simulink model "twolevel_seriesparallel"  (R2016a)
settings: Solver=VariableStepAuto  StartTime=0.0  StopTime=stop_time  RelTol=1e-3  AbsTol=1e-6
values from neighbouring files (symbols this model uses):
  DCLINK_Cap = 0.65*1.35*capacitorsabiti/sw_frequency    (= 0.000406115702479)    [loadvariation.m]    (also in trials.m = 1.35*capacitorsabiti/sw_frequency; twolevel_seriesparallel_analysis.m)
  Ef = Vln_rms*cos(Load_Angle)    [loadvariation.m]    (also in trials.m; twolevel_seriesparallel_analysis.m)
  intangle1 = 0    [loadvariation.m]    (also in trials.m; twolevel_seriesparallel_analysis.m)
  intangle2 = interleaving_angle    (= 180)    [loadvariation.m]    (also in trials.m = 360; twolevel_seriesparallel_analysis.m)
  intangle3 = 0    [loadvariation.m]    (also in trials.m; twolevel_seriesparallel_analysis.m)
  intangle4 = interleaving_angle    (= 180)    [loadvariation.m]    (also in trials.m = 360; twolevel_seriesparallel_analysis.m)
  Load_Angle = acos(Load_Power_Factor)    [loadvariation.m]    (also in trials.m; twolevel_seriesparallel_analysis.m)
  Ls = n*m*Xs/ref_frequency    [loadvariation.m]    (also in trials.m; twolevel_seriesparallel_analysis.m)
  ma = 0.9    [loadvariation.m]    (also in trials.m; twolevel_seriesparallel_analysis.m)
  ref_frequency = 2*pi*50    (= 314.159265359)    [loadvariation.m]    (also in trials.m; twolevel_seriesparallel_analysis.m)
  Sampling_time = 1/(100*sw_frequency)    (= 1.65289256198e-06)    [loadvariation.m]    (also in twolevel_seriesparallel_analysis.m = 8.26446280992e-06)
  Vin = DC_Voltage_Source + Rin*(Load_Real_Power/DC_Voltage_Source)    (= 554.814814815)    [loadvariation.m]    (also in trials.m; twolevel_seriesparallel_analysis.m)
undefined symbols (not defined in the file or in its folder): intangle5, intangle6, intangle7, intangle8, Lload, Rload
libraries: powerlib x106, powerlib_meascontrol x58, simulink x24
(part 1 of 2)
settings Model: Creator=hakan  LastModifiedBy=hakan
settings DataIOCC: SaveState=on
settings DebuggingCC: UnconnectedInputMsg=none  UnconnectedOutputMsg=none  UnconnectedLineMsg=none

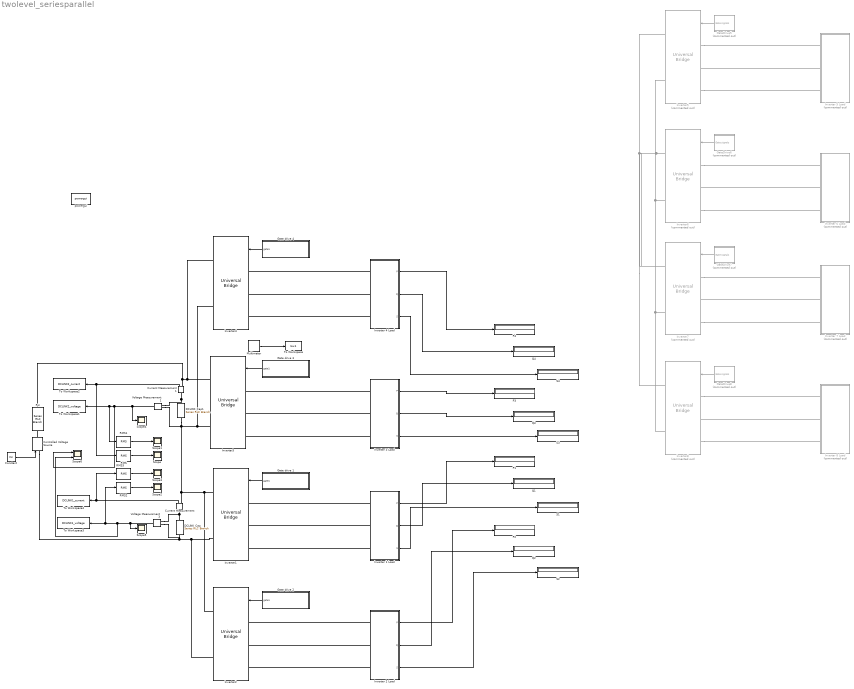
== system twolevel_seriesparallel ==
  Constant : Constant  Value=Vin
  Controlled Voltage Source : powerlib/Electrical Sources/Controlled Voltage Source  Initialize=on  Source_Type=AC  Amplitude=0  Phase=0  Frequency=0  Measurements=None
  Current Measurement : powerlib/Measurements/Current Measurement  PhasorSimulation=off  OutputType=Complex  PSBequivalent=0
  Current Measurement1 : powerlib/Measurements/Current Measurement  PhasorSimulation=off  OutputType=Complex  PSBequivalent=0
  DCLINK_Cap : powerlib/Elements/Series RLC Branch  LConnTagsString=__new0  RConnTagsString=__new0  BranchType=C  Resistance=1  Inductance=1e-3  SetiL0=off  InitialCurrent=0  Capacitance=DCLINK_Cap  Setx0=on  InitialVoltage=270  Measurements=None
  DCLINK_Cap1 : powerlib/Elements/Series RLC Branch  LConnTagsString=__new0  RConnTagsString=__new0  BranchType=C  Resistance=1  Inductance=1e-3  SetiL0=off  InitialCurrent=0  Capacitance=DCLINK_Cap  Setx0=on  InitialVoltage=270  Measurements=None
  Gate drive 1 : Subsystem
  Gate drive 2 : Subsystem
  Gate drive 3 : Subsystem
  Gate drive 4 : Subsystem
  GateDrive5 : Subsystem  Commented=on
  GateDrive6 : Subsystem  Commented=on
  GateDrive7 : Subsystem  Commented=on
  GateDrive8 : Subsystem  Commented=on
  Inverter 1 Load : Subsystem
  Inverter 2 Load : Subsystem
  Inverter 3 Load : Subsystem
  Inverter 4 Load : Subsystem
  Inverter 5 Load : Subsystem  Commented=on
  Inverter 6 Load : Subsystem  Commented=on
  Inverter 7 Load : Subsystem  Commented=on
  Inverter 8 Load : Subsystem  Commented=on
  Inverter1 : powerlib/Power Electronics/Universal Bridge  Arms=3  SnubberResistance=1e5  SnubberCapacitance=inf  Device=IGBT / Diodes  Ron=1e-3  Lon=0  ForwardVoltages="[  0  0  ]"  ForwardVoltage=0  GTOparameters=[ 10e-6 , 20e-6 ]  IGBTparameters=[ 1e-6 , 2e-6 ]  Measurements=None  Measurements_2=None  converterType=Rectifier
  Inverter2 : powerlib/Power Electronics/Universal Bridge  Arms=3  SnubberResistance=1e5  SnubberCapacitance=inf  Device=IGBT / Diodes  Ron=1e-3  Lon=0  ForwardVoltages="[  0  0  ]"  ForwardVoltage=0  GTOparameters=[ 10e-6 , 20e-6 ]  IGBTparameters=[ 1e-6 , 2e-6 ]  Measurements=None  Measurements_2=None  converterType=Rectifier
  Inverter3 : powerlib/Power Electronics/Universal Bridge  Arms=3  SnubberResistance=1e5  SnubberCapacitance=inf  Device=IGBT / Diodes  Ron=1e-3  Lon=0  ForwardVoltages="[  0  0  ]"  ForwardVoltage=0  GTOparameters=[ 10e-6 , 20e-6 ]  IGBTparameters=[ 1e-6 , 2e-6 ]  Measurements=All voltages and currents  Measurements_2=None  converterType=Rectifier
  Inverter4 : powerlib/Power Electronics/Universal Bridge  Arms=3  SnubberResistance=1e5  SnubberCapacitance=inf  Device=IGBT / Diodes  Ron=1e-3  Lon=0  ForwardVoltages="[  0  0  ]"  ForwardVoltage=0  GTOparameters=[ 10e-6 , 20e-6 ]  IGBTparameters=[ 1e-6 , 2e-6 ]  Measurements=None  Measurements_2=None  converterType=Rectifier
  Inverter{5..8} (4 alike) : powerlib/Power Electronics/Universal Bridge  Commented=on  Arms=3  SnubberResistance=1e5  SnubberCapacitance=inf  Device=IGBT / Diodes  Ron=1e-3  Lon=0  ForwardVoltages="[  0  0  ]"  ForwardVoltage=0  GTOparameters=[ 10e-6 , 20e-6 ]  IGBTparameters=[ 1e-6 , 2e-6 ]  Measurements=None  Measurements_2=None  converterType=Rectifier
  Multimeter : powerlib/Measurements/Multimeter  PhasorSimulation=off  OutputType=Complex  sel=11  L=16  Gain=1  yselected={'Isw1: Inverter3'};  PSBOutputType=1  PSBequivalent=0  AxesSetting=[0,0.1,-100,100]  Display=0  SavedBlockNames=-11
  P{1..4} (4 alike) : Display
  Q{1..4} (4 alike) : Display
  RMS{,1..3} (4 alike) : powerlib_meascontrol/Measurements/RMS  TrueRMS=on  Freq=Load_Nominal_Freq  RMSInit=10  Ts=0
  Rin : powerlib/Elements/Series RLC Branch  LConnTagsString=__new0  RConnTagsString=__new0  BranchType=R  Resistance=1  Inductance=1e-3  SetiL0=off  InitialCurrent=0  Capacitance=1000e-6  Setx0=off  InitialVoltage=0  Measurements=None
  S{1..4} (4 alike) : Display
  Scope{,1..5} (6 alike) : Scope
  Scope6 : Scope  NumInputPorts=2
  To Workspace : ToWorkspace  VariableName=Isw1  SaveFormat=Structure With Time  SampleTime=-1
  To Workspace1 : ToWorkspace  VariableName=DCLINK2_voltage  SaveFormat=Structure With Time  SampleTime=-1
  To Workspace2 : ToWorkspace  VariableName=DCLINK2_current  SaveFormat=Structure With Time  SampleTime=-1
  To Workspace3 : ToWorkspace  VariableName=DCLINK1_voltage  SaveFormat=Structure With Time  SampleTime=-1
  To Workspace4 : ToWorkspace  VariableName=DCLINK1_current  SaveFormat=Structure With Time  SampleTime=-1
  Voltage Measurement1 : powerlib/Measurements/Voltage Measurement  PhasorSimulation=off  OutputType=Complex  PSBequivalent=0
  Voltage Measurement3 : powerlib/Measurements/Voltage Measurement  PhasorSimulation=off  OutputType=Complex  PSBequivalent=0
  powergui : powerlib/powergui  Priority=1  SimulationMode=Discrete  SolverType=Tustin/Backward Euler (TBE)  SampleTime=Sampling_time  frequency=60  SPID=off  DisableSnubberDevices=off  DisableRonSwitches=off  DisableVfSwitches=off  SwTol=0  DisplayEquations=off  Interpol=off  ExternalGateDelay=off  methode=off  Ts=10  FunctionMessages=off  echomessages=off  HookPort=off  EnableUseOfTLC=off  x0status=blocks  frequencyindice=0  Pbase=100e6  ErrMax=1e-4  Iterations=50  UnitsV=kV  UnitsW=MW  buscounter=0  RestoreLinks=warning  ResistiveCurrentMeasurement=off  Frange=[0:2:500]  Ylog=off  Xlog=on  ShowGrid=off  save=off  variable=ZData  structure=DCLINK1_current  ZoomFFT=off  StartTime=0  cycles=35  DisplayStyle=4  fundamental=50  FreqAxis=off  MaxFrequency=300000  frequencyindicesteady=1  RmsSteady=1  display=off
  wires:
  Constant/1 -> Controlled Voltage Source/1
  Gate drive 1/1(gate1) -> Inverter1/1
  Current Measurement/1 -> RMS3/1, To Workspace4/1
  Gate drive 2/1(gate1) -> Inverter2/1
  GateDrive5/1(Gate signals) -> Inverter5/1
  GateDrive6/1(Gate signals) -> Inverter6/1
  GateDrive7/1(Gate signals) -> Inverter7/1
  GateDrive8/1(Gate signals) -> Inverter8/1
  Current Measurement1/1 -> RMS/1, To Workspace2/1
  Voltage Measurement1/1 -> Scope4/1, Scope6/1, RMS1/1, To Workspace1/1
  RMS/1 -> Scope/1
  RMS1/1 -> Scope1/1
  RMS2/1 -> Scope2/1
  RMS3/1 -> Scope3/1
  Voltage Measurement3/1 -> Scope6/2, RMS2/1, To Workspace3/1, Scope5/1
  Gate drive 4/1(gate1) -> Inverter4/1
  Gate drive 3/1(gate1) -> Inverter3/1
  Inverter 1 Load/2(Q) -> Q1/1
  Inverter 1 Load/3(S) -> S1/1
  Inverter 2 Load/1(P) -> P2/1
  Inverter 2 Load/2(Q) -> Q2/1
  Inverter 2 Load/3(S) -> S2/1
  Inverter 1 Load/1(P) -> P1/1
  Inverter 4 Load/2(Q) -> Q4/1
  Inverter 4 Load/3(S) -> S4/1
  Inverter 3 Load/1(P) -> P3/1
  Inverter 3 Load/2(Q) -> Q3/1
  Inverter 3 Load/3(S) -> S3/1
  Inverter 4 Load/1(P) -> P4/1
  Multimeter/1 -> To Workspace/1
  connections:
  Voltage Measurement3/LConn1 -- Current Measurement/LConn1 -- DCLINK_Cap/LConn1
  Inverter 1 Load/LConn3 -- Inverter1/LConn3
  Inverter 1 Load/LConn1 -- Inverter1/LConn1
  Controlled Voltage Source/RConn1 -- Rin/RConn1
  Inverter 2 Load/LConn2 -- Inverter2/LConn2
  Inverter 1 Load/LConn2 -- Inverter1/LConn2
  Inverter 2 Load/LConn1 -- Inverter2/LConn1
  Inverter 2 Load/LConn3 -- Inverter2/LConn3
  Inverter 3 Load/LConn1 -- Inverter3/LConn1
  Inverter 4 Load/LConn3 -- Inverter4/LConn3
  Inverter 3 Load/LConn3 -- Inverter3/LConn3
  Inverter 3 Load/LConn2 -- Inverter3/LConn2
  Inverter 4 Load/LConn1 -- Inverter4/LConn1
  Inverter 4 Load/LConn2 -- Inverter4/LConn2
  Inverter7/LConn3 -- Inverter 7 Load/LConn3
  Inverter6/LConn3 -- Inverter 6 Load/LConn3
  Inverter5/LConn1 -- Inverter 5 Load/LConn1
  Inverter 5 Load/LConn2 -- Inverter5/LConn2
  Inverter8/LConn3 -- Inverter 8 Load/LConn3
  Inverter5/LConn3 -- Inverter 5 Load/LConn3
  Inverter7/LConn1 -- Inverter 7 Load/LConn1
  Inverter6/LConn1 -- Inverter 6 Load/LConn1
  Inverter 8 Load/LConn2 -- Inverter8/LConn2
  Inverter 6 Load/LConn2 -- Inverter6/LConn2
  Inverter8/LConn1 -- Inverter 8 Load/LConn1
  Inverter 7 Load/LConn2 -- Inverter7/LConn2
  DCLINK_Cap1/LConn1 -- Current Measurement1/LConn1 -- Voltage Measurement1/LConn1
  Inverter8/RConn2 -- Inverter5/RConn2 -- Inverter6/RConn2 -- Inverter7/RConn2
  Inverter6/RConn1 -- Inverter8/RConn1 -- Inverter7/RConn1 -- Inverter5/RConn1
  Current Measurement1/RConn1 -- Rin/LConn1 -- Inverter4/RConn1 -- Inverter3/RConn1
  Inverter2/RConn2 -- Inverter1/RConn2 -- Controlled Voltage Source/LConn1 -- DCLINK_Cap/RConn1 -- Voltage Measurement3/LConn2
  Voltage Measurement1/LConn2 -- Inverter4/RConn2 -- Inverter3/RConn2 -- DCLINK_Cap1/RConn1 -- Current Measurement/RConn1 -- Inverter2/RConn1 -- Inverter1/RConn1

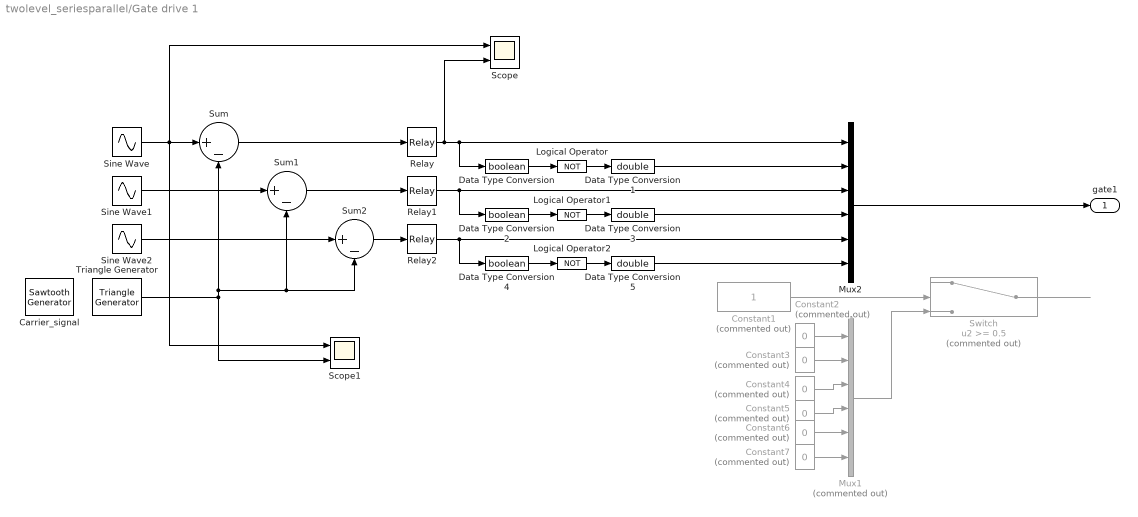
== system twolevel_seriesparallel/Gate drive 1 ==
  Carrier_signal : powerlib_meascontrol/Pulse & Signal Generators/Sawtooth Generator  Freq=sw_frequency  Phase=intangle1  Ts=0
  Constant1 : Constant  Commented=on
  Constant{2..7} (6 alike) : Constant  Commented=on  Value=0
  Data Type Conversion : DataTypeConversion  OutDataTypeStr=boolean
  Data Type Conversion1 : DataTypeConversion  OutDataTypeStr=double
  Data Type Conversion2 : DataTypeConversion  OutDataTypeStr=boolean
  Data Type Conversion3 : DataTypeConversion  OutDataTypeStr=double
  Data Type Conversion4 : DataTypeConversion  OutDataTypeStr=boolean
  Data Type Conversion5 : DataTypeConversion  OutDataTypeStr=double
  Logical Operator : Logic  Operator=NOT  AllPortsSameDT=off  OutDataTypeStr=boolean
  Logical Operator1 : Logic  Operator=NOT  AllPortsSameDT=off  OutDataTypeStr=boolean
  Logical Operator2 : Logic  Operator=NOT  AllPortsSameDT=off  OutDataTypeStr=boolean
  Mux1 : Mux  Commented=on  Inputs=6
  Mux2 : Mux  Inputs=6
  Relay : Relay
  Relay1 : Relay
  Relay2 : Relay
  Scope : Scope  NumInputPorts=2
  Scope1 : Scope  NumInputPorts=2
  Sine Wave : Sin  Amplitude=ma  Frequency=ref_frequency  Phase=Load_Angle  SampleTime=0
  Sine Wave1 : Sin  Amplitude=ma  Frequency=ref_frequency  Phase=-2*pi/3+Load_Angle  SampleTime=0
  Sine Wave2 : Sin  Amplitude=ma  Frequency=ref_frequency  Phase=2*pi/3+Load_Angle  SampleTime=0
  Sum : Sum  Inputs=|+-
  Sum1 : Sum  Inputs=|+-
  Sum2 : Sum  Inputs=|+-
  Switch : Switch  Commented=on  Threshold=0.5
  Triangle Generator : powerlib_meascontrol/Pulse & Signal Generators/Triangle Generator  Freq=sw_frequency  Phase=intangle1  Ts=0
  gate1 : Outport
  wires:
  Sine Wave/1 -> Scope1/1, Scope/1, Sum/1
  Triangle Generator/1 -> Sum1/2, Sum2/2, Sum/2, Scope1/2
  Sine Wave1/1 -> Sum1/1
  Sine Wave2/1 -> Sum2/1
  Sum/1 -> Relay/1
  Sum1/1 -> Relay1/1
  Sum2/1 -> Relay2/1
  Data Type Conversion/1 -> Logical Operator/1
  Relay/1 -> Scope/2, Data Type Conversion/1, Mux2/1
  Logical Operator/1 -> Data Type Conversion1/1
  Data Type Conversion1/1 -> Mux2/2
  Data Type Conversion2/1 -> Logical Operator1/1
  Relay1/1 -> Data Type Conversion2/1, Mux2/3
  Logical Operator1/1 -> Data Type Conversion3/1
  Data Type Conversion3/1 -> Mux2/4
  Data Type Conversion4/1 -> Logical Operator2/1
  Relay2/1 -> Data Type Conversion4/1, Mux2/5
  Logical Operator2/1 -> Data Type Conversion5/1
  Data Type Conversion5/1 -> Mux2/6
  Constant1/1 -> Switch/2
  Constant2/1 -> Mux1/1
  Constant3/1 -> Mux1/2
  Constant4/1 -> Mux1/3
  Constant5/1 -> Mux1/4
  Constant7/1 -> Mux1/6
  Constant6/1 -> Mux1/5
  Mux1/1 -> Switch/3
  Switch/1 -> ?
  Mux2/1 -> gate1/1

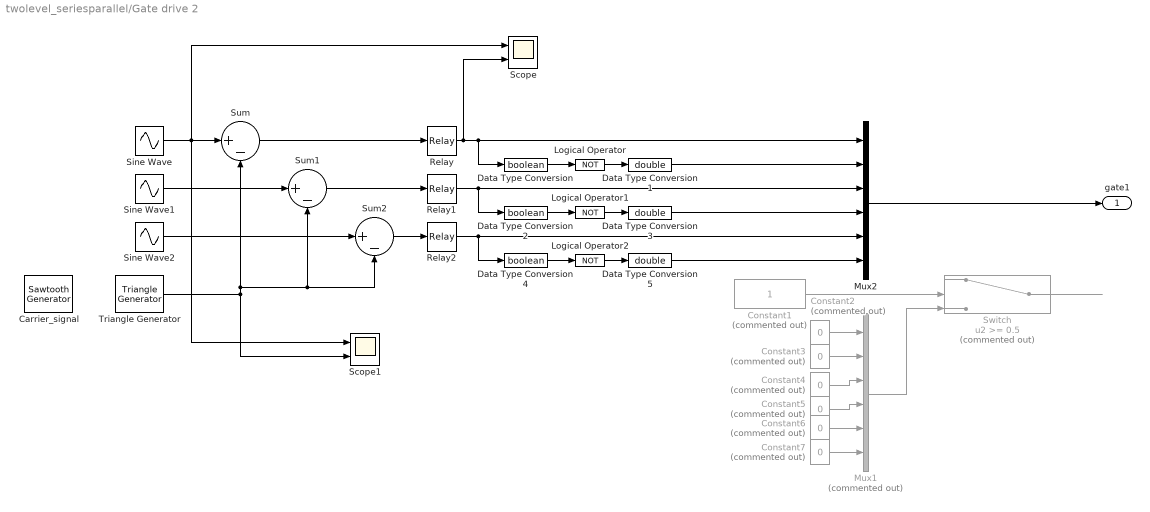
== system twolevel_seriesparallel/Gate drive 2 ==
  Carrier_signal : powerlib_meascontrol/Pulse & Signal Generators/Sawtooth Generator  Freq=sw_frequency  Phase=intangle2  Ts=0
  Constant1 : Constant  Commented=on
  Constant{2..7} (6 alike) : Constant  Commented=on  Value=0
  Data Type Conversion : DataTypeConversion  OutDataTypeStr=boolean
  Data Type Conversion1 : DataTypeConversion  OutDataTypeStr=double
  Data Type Conversion2 : DataTypeConversion  OutDataTypeStr=boolean
  Data Type Conversion3 : DataTypeConversion  OutDataTypeStr=double
  Data Type Conversion4 : DataTypeConversion  OutDataTypeStr=boolean
  Data Type Conversion5 : DataTypeConversion  OutDataTypeStr=double
  Logical Operator : Logic  Operator=NOT  AllPortsSameDT=off  OutDataTypeStr=boolean
  Logical Operator1 : Logic  Operator=NOT  AllPortsSameDT=off  OutDataTypeStr=boolean
  Logical Operator2 : Logic  Operator=NOT  AllPortsSameDT=off  OutDataTypeStr=boolean
  Mux1 : Mux  Commented=on  Inputs=6
  Mux2 : Mux  Inputs=6
  Relay : Relay
  Relay1 : Relay
  Relay2 : Relay
  Scope : Scope  NumInputPorts=2
  Scope1 : Scope  NumInputPorts=2
  Sine Wave : Sin  Amplitude=ma  Frequency=ref_frequency  Phase=Load_Angle  SampleTime=0
  Sine Wave1 : Sin  Amplitude=ma  Frequency=ref_frequency  Phase=-2*pi/3+Load_Angle  SampleTime=0
  Sine Wave2 : Sin  Amplitude=ma  Frequency=ref_frequency  Phase=2*pi/3+Load_Angle  SampleTime=0
  Sum : Sum  Inputs=|+-
  Sum1 : Sum  Inputs=|+-
  Sum2 : Sum  Inputs=|+-
  Switch : Switch  Commented=on  Threshold=0.5
  Triangle Generator : powerlib_meascontrol/Pulse & Signal Generators/Triangle Generator  Freq=sw_frequency  Phase=intangle2  Ts=0
  gate1 : Outport
  wires:
  Sine Wave/1 -> Scope1/1, Scope/1, Sum/1
  Triangle Generator/1 -> Sum1/2, Sum2/2, Sum/2, Scope1/2
  Sine Wave1/1 -> Sum1/1
  Sine Wave2/1 -> Sum2/1
  Sum/1 -> Relay/1
  Sum1/1 -> Relay1/1
  Sum2/1 -> Relay2/1
  Data Type Conversion/1 -> Logical Operator/1
  Relay/1 -> Scope/2, Data Type Conversion/1, Mux2/1
  Logical Operator/1 -> Data Type Conversion1/1
  Data Type Conversion1/1 -> Mux2/2
  Data Type Conversion2/1 -> Logical Operator1/1
  Relay1/1 -> Data Type Conversion2/1, Mux2/3
  Logical Operator1/1 -> Data Type Conversion3/1
  Data Type Conversion3/1 -> Mux2/4
  Data Type Conversion4/1 -> Logical Operator2/1
  Relay2/1 -> Data Type Conversion4/1, Mux2/5
  Logical Operator2/1 -> Data Type Conversion5/1
  Data Type Conversion5/1 -> Mux2/6
  Constant1/1 -> Switch/2
  Constant2/1 -> Mux1/1
  Constant3/1 -> Mux1/2
  Constant4/1 -> Mux1/3
  Constant5/1 -> Mux1/4
  Constant7/1 -> Mux1/6
  Constant6/1 -> Mux1/5
  Mux1/1 -> Switch/3
  Switch/1 -> ?
  Mux2/1 -> gate1/1

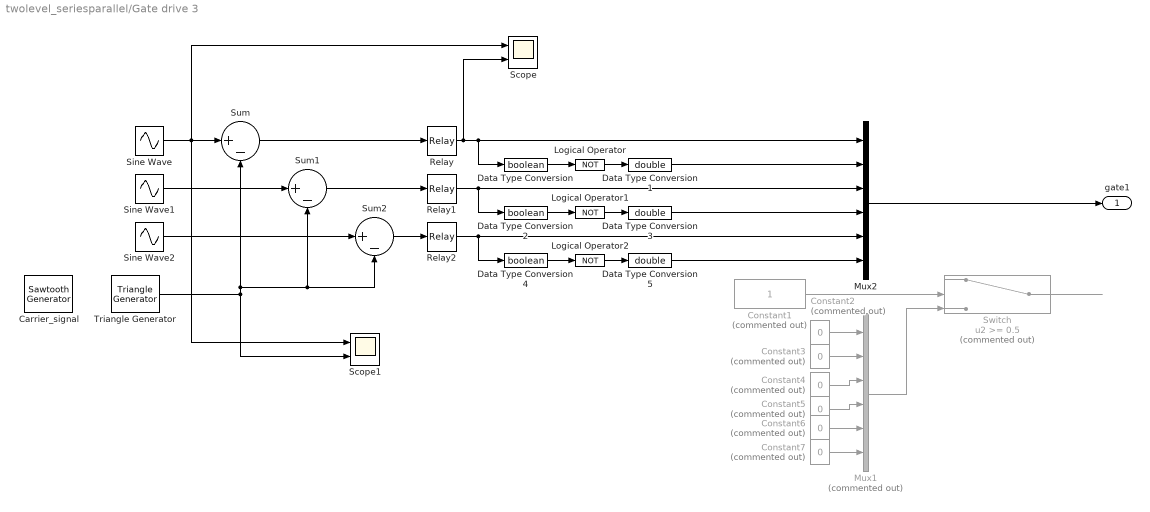
== system twolevel_seriesparallel/Gate drive 3 ==
  Carrier_signal : powerlib_meascontrol/Pulse & Signal Generators/Sawtooth Generator  Freq=sw_frequency  Phase=intangle3  Ts=0
  Constant1 : Constant  Commented=on
  Constant{2..7} (6 alike) : Constant  Commented=on  Value=0
  Data Type Conversion : DataTypeConversion  OutDataTypeStr=boolean
  Data Type Conversion1 : DataTypeConversion  OutDataTypeStr=double
  Data Type Conversion2 : DataTypeConversion  OutDataTypeStr=boolean
  Data Type Conversion3 : DataTypeConversion  OutDataTypeStr=double
  Data Type Conversion4 : DataTypeConversion  OutDataTypeStr=boolean
  Data Type Conversion5 : DataTypeConversion  OutDataTypeStr=double
  Logical Operator : Logic  Operator=NOT  AllPortsSameDT=off  OutDataTypeStr=boolean
  Logical Operator1 : Logic  Operator=NOT  AllPortsSameDT=off  OutDataTypeStr=boolean
  Logical Operator2 : Logic  Operator=NOT  AllPortsSameDT=off  OutDataTypeStr=boolean
  Mux1 : Mux  Commented=on  Inputs=6
  Mux2 : Mux  Inputs=6
  Relay : Relay
  Relay1 : Relay
  Relay2 : Relay
  Scope : Scope  NumInputPorts=2
  Scope1 : Scope  NumInputPorts=2
  Sine Wave : Sin  Amplitude=ma  Frequency=ref_frequency  Phase=Load_Angle  SampleTime=0
  Sine Wave1 : Sin  Amplitude=ma  Frequency=ref_frequency  Phase=-2*pi/3+Load_Angle  SampleTime=0
  Sine Wave2 : Sin  Amplitude=ma  Frequency=ref_frequency  Phase=2*pi/3+Load_Angle  SampleTime=0
  Sum : Sum  Inputs=|+-
  Sum1 : Sum  Inputs=|+-
  Sum2 : Sum  Inputs=|+-
  Switch : Switch  Commented=on  Threshold=0.5
  Triangle Generator : powerlib_meascontrol/Pulse & Signal Generators/Triangle Generator  Freq=sw_frequency  Phase=intangle3  Ts=0
  gate1 : Outport
  wires:
  Mux2/1 -> gate1/1
  Switch/1 -> ?
  Mux1/1 -> Switch/3
  Constant6/1 -> Mux1/5
  Constant7/1 -> Mux1/6
  Constant5/1 -> Mux1/4
  Constant4/1 -> Mux1/3
  Constant3/1 -> Mux1/2
  Constant2/1 -> Mux1/1
  Constant1/1 -> Switch/2
  Data Type Conversion5/1 -> Mux2/6
  Logical Operator2/1 -> Data Type Conversion5/1
  Relay2/1 -> Mux2/5, Data Type Conversion4/1
  Data Type Conversion4/1 -> Logical Operator2/1
  Data Type Conversion3/1 -> Mux2/4
  Logical Operator1/1 -> Data Type Conversion3/1
  Relay1/1 -> Mux2/3, Data Type Conversion2/1
  Data Type Conversion2/1 -> Logical Operator1/1
  Data Type Conversion1/1 -> Mux2/2
  Logical Operator/1 -> Data Type Conversion1/1
  Relay/1 -> Mux2/1, Data Type Conversion/1, Scope/2
  Data Type Conversion/1 -> Logical Operator/1
  Sum2/1 -> Relay2/1
  Sum1/1 -> Relay1/1
  Sum/1 -> Relay/1
  Sine Wave2/1 -> Sum2/1
  Sine Wave1/1 -> Sum1/1
  Triangle Generator/1 -> Scope1/2, Sum/2, Sum2/2, Sum1/2
  Sine Wave/1 -> Sum/1, Scope/1, Scope1/1

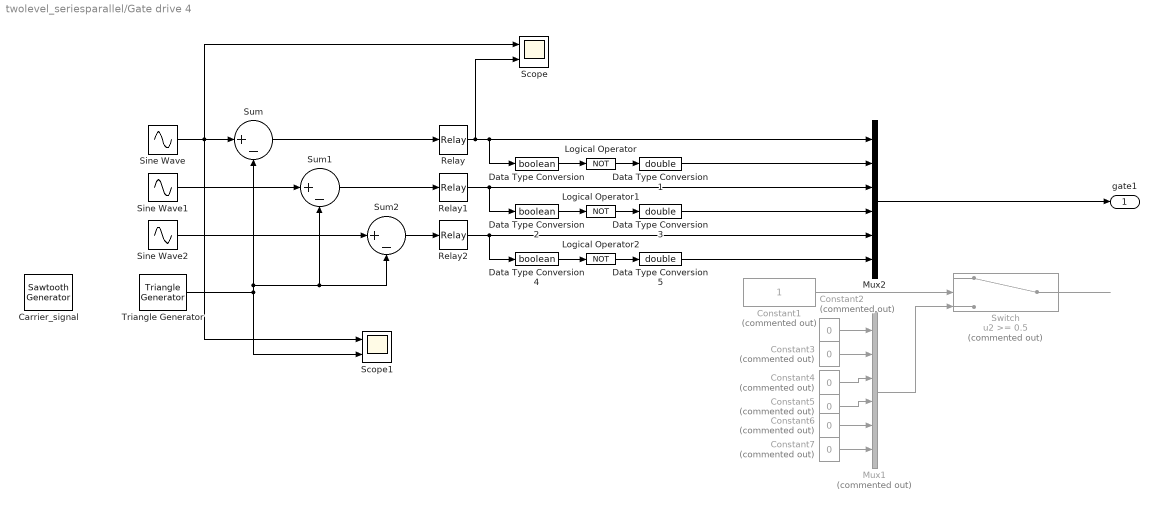
== system twolevel_seriesparallel/Gate drive 4 ==
  Carrier_signal : powerlib_meascontrol/Pulse & Signal Generators/Sawtooth Generator  Freq=sw_frequency  Phase=intangle4  Ts=0
  Constant1 : Constant  Commented=on
  Constant{2..7} (6 alike) : Constant  Commented=on  Value=0
  Data Type Conversion : DataTypeConversion  OutDataTypeStr=boolean
  Data Type Conversion1 : DataTypeConversion  OutDataTypeStr=double
  Data Type Conversion2 : DataTypeConversion  OutDataTypeStr=boolean
  Data Type Conversion3 : DataTypeConversion  OutDataTypeStr=double
  Data Type Conversion4 : DataTypeConversion  OutDataTypeStr=boolean
  Data Type Conversion5 : DataTypeConversion  OutDataTypeStr=double
  Logical Operator : Logic  Operator=NOT  AllPortsSameDT=off  OutDataTypeStr=boolean
  Logical Operator1 : Logic  Operator=NOT  AllPortsSameDT=off  OutDataTypeStr=boolean
  Logical Operator2 : Logic  Operator=NOT  AllPortsSameDT=off  OutDataTypeStr=boolean
  Mux1 : Mux  Commented=on  Inputs=6
  Mux2 : Mux  Inputs=6
  Relay : Relay
  Relay1 : Relay
  Relay2 : Relay
  Scope : Scope  NumInputPorts=2
  Scope1 : Scope  NumInputPorts=2
  Sine Wave : Sin  Amplitude=ma  Frequency=ref_frequency  Phase=Load_Angle  SampleTime=0
  Sine Wave1 : Sin  Amplitude=ma  Frequency=ref_frequency  Phase=-2*pi/3+Load_Angle  SampleTime=0
  Sine Wave2 : Sin  Amplitude=ma  Frequency=ref_frequency  Phase=2*pi/3+Load_Angle  SampleTime=0
  Sum : Sum  Inputs=|+-
  Sum1 : Sum  Inputs=|+-
  Sum2 : Sum  Inputs=|+-
  Switch : Switch  Commented=on  Threshold=0.5
  Triangle Generator : powerlib_meascontrol/Pulse & Signal Generators/Triangle Generator  Freq=sw_frequency  Phase=intangle4  Ts=0
  gate1 : Outport
  wires:
  Sine Wave/1 -> Scope1/1, Scope/1, Sum/1
  Triangle Generator/1 -> Sum1/2, Sum2/2, Sum/2, Scope1/2
  Sine Wave1/1 -> Sum1/1
  Sine Wave2/1 -> Sum2/1
  Sum/1 -> Relay/1
  Sum1/1 -> Relay1/1
  Sum2/1 -> Relay2/1
  Data Type Conversion/1 -> Logical Operator/1
  Relay/1 -> Scope/2, Data Type Conversion/1, Mux2/1
  Logical Operator/1 -> Data Type Conversion1/1
  Data Type Conversion1/1 -> Mux2/2
  Data Type Conversion2/1 -> Logical Operator1/1
  Relay1/1 -> Data Type Conversion2/1, Mux2/3
  Logical Operator1/1 -> Data Type Conversion3/1
  Data Type Conversion3/1 -> Mux2/4
  Data Type Conversion4/1 -> Logical Operator2/1
  Relay2/1 -> Data Type Conversion4/1, Mux2/5
  Logical Operator2/1 -> Data Type Conversion5/1
  Data Type Conversion5/1 -> Mux2/6
  Constant1/1 -> Switch/2
  Constant2/1 -> Mux1/1
  Constant3/1 -> Mux1/2
  Constant4/1 -> Mux1/3
  Constant5/1 -> Mux1/4
  Constant7/1 -> Mux1/6
  Constant6/1 -> Mux1/5
  Mux1/1 -> Switch/3
  Switch/1 -> ?
  Mux2/1 -> gate1/1

== system twolevel_seriesparallel/GateDrive5 ==
  Bus Creator : BusCreator  Inputs=6
  Carrier_signal : powerlib_meascontrol/Pulse & Signal Generators/Sawtooth Generator  Freq=sw_frequency  Phase=intangle5  Ts=0
  Compare To Zero : simulink/Logic and Bit Operations/Compare To Zero  relop=>=  OutDataTypeStr=boolean  ZeroCross=off
  Compare To Zero1 : simulink/Logic and Bit Operations/Compare To Zero  relop=>=  OutDataTypeStr=boolean  ZeroCross=off
  Compare To Zero2 : simulink/Logic and Bit Operations/Compare To Zero  relop=>=  OutDataTypeStr=boolean  ZeroCross=off
  Compare To Zero3 : simulink/Logic and Bit Operations/Compare To Zero  relop===  OutDataTypeStr=boolean  ZeroCross=off
  Compare To Zero4 : simulink/Logic and Bit Operations/Compare To Zero  relop===  OutDataTypeStr=boolean  ZeroCross=off
  Compare To Zero5 : simulink/Logic and Bit Operations/Compare To Zero  relop===  OutDataTypeStr=boolean  ZeroCross=off
  PhaseA_Ref : Sin  Amplitude=ma  Frequency=ref_frequency  SampleTime=0
  PhaseB_Ref : Sin  Amplitude=ma  Frequency=ref_frequency  Phase=-2*pi/3  SampleTime=0
  PhaseC_Ref : Sin  Amplitude=ma  Frequency=ref_frequency  Phase=2*pi/3  SampleTime=0
  Sum1 : Sum  Inputs=|+-
  Sum2 : Sum  Inputs=|+-
  Sum3 : Sum  Inputs=|+-
  Gate signals : Outport
  wires:
  Bus Creator/1 -> Gate signals/1
  PhaseA_Ref/1 -> Sum2/1
  Compare To Zero/1 -> Compare To Zero3/1, Bus Creator/1
  Sum2/1 -> Compare To Zero/1
  [Carrier] -> Sum2/2
  Compare To Zero1/1 -> Compare To Zero4/1, Bus Creator/3
  PhaseB_Ref/1 -> Sum1/1
  [Carrier] -> Sum1/2
  Compare To Zero2/1 -> Compare To Zero5/1, Bus Creator/5
  PhaseC_Ref/1 -> Sum3/1
  [Carrier] -> Sum3/2
  Sum1/1 -> Compare To Zero1/1
  Sum3/1 -> Compare To Zero2/1
  Compare To Zero3/1 -> Bus Creator/2
  Compare To Zero4/1 -> Bus Creator/4
  Compare To Zero5/1 -> Bus Creator/6
  Carrier_signal/1 -> [Carrier]

== system twolevel_seriesparallel/GateDrive6 ==
  Bus Creator : BusCreator  Inputs=6
  Carrier_signal : powerlib_meascontrol/Pulse & Signal Generators/Sawtooth Generator  Freq=sw_frequency  Phase=intangle6  Ts=0
  Compare To Zero : simulink/Logic and Bit Operations/Compare To Zero  relop=>=  OutDataTypeStr=boolean  ZeroCross=off
  Compare To Zero1 : simulink/Logic and Bit Operations/Compare To Zero  relop=>=  OutDataTypeStr=boolean  ZeroCross=off
  Compare To Zero2 : simulink/Logic and Bit Operations/Compare To Zero  relop=>=  OutDataTypeStr=boolean  ZeroCross=off
  Compare To Zero3 : simulink/Logic and Bit Operations/Compare To Zero  relop===  OutDataTypeStr=boolean  ZeroCross=off
  Compare To Zero4 : simulink/Logic and Bit Operations/Compare To Zero  relop===  OutDataTypeStr=boolean  ZeroCross=off
  Compare To Zero5 : simulink/Logic and Bit Operations/Compare To Zero  relop===  OutDataTypeStr=boolean  ZeroCross=off
  PhaseA_Ref : Sin  Amplitude=ma  Frequency=ref_frequency  SampleTime=0
  PhaseB_Ref : Sin  Amplitude=ma  Frequency=ref_frequency  Phase=-2*pi/3  SampleTime=0
  PhaseC_Ref : Sin  Amplitude=ma  Frequency=ref_frequency  Phase=2*pi/3  SampleTime=0
  Sum1 : Sum  Inputs=|+-
  Sum2 : Sum  Inputs=|+-
  Sum3 : Sum  Inputs=|+-
  Gate signals : Outport
  wires:
  Carrier_signal/1 -> [Carrier]
  Compare To Zero5/1 -> Bus Creator/6
  Compare To Zero4/1 -> Bus Creator/4
  Compare To Zero3/1 -> Bus Creator/2
  Sum3/1 -> Compare To Zero2/1
  Sum1/1 -> Compare To Zero1/1
  [Carrier] -> Sum3/2
  PhaseC_Ref/1 -> Sum3/1
  Compare To Zero2/1 -> Bus Creator/5, Compare To Zero5/1
  [Carrier] -> Sum1/2
  PhaseB_Ref/1 -> Sum1/1
  Compare To Zero1/1 -> Bus Creator/3, Compare To Zero4/1
  [Carrier] -> Sum2/2
  Sum2/1 -> Compare To Zero/1
  Compare To Zero/1 -> Bus Creator/1, Compare To Zero3/1
  PhaseA_Ref/1 -> Sum2/1
  Bus Creator/1 -> Gate signals/1

== system twolevel_seriesparallel/GateDrive7 ==
  Bus Creator : BusCreator  Inputs=6
  Carrier_signal : powerlib_meascontrol/Pulse & Signal Generators/Sawtooth Generator  Freq=sw_frequency  Phase=intangle7  Ts=0
  Compare To Zero : simulink/Logic and Bit Operations/Compare To Zero  relop=>=  OutDataTypeStr=boolean  ZeroCross=off
  Compare To Zero1 : simulink/Logic and Bit Operations/Compare To Zero  relop=>=  OutDataTypeStr=boolean  ZeroCross=off
  Compare To Zero2 : simulink/Logic and Bit Operations/Compare To Zero  relop=>=  OutDataTypeStr=boolean  ZeroCross=off
  Compare To Zero3 : simulink/Logic and Bit Operations/Compare To Zero  relop===  OutDataTypeStr=boolean  ZeroCross=off
  Compare To Zero4 : simulink/Logic and Bit Operations/Compare To Zero  relop===  OutDataTypeStr=boolean  ZeroCross=off
  Compare To Zero5 : simulink/Logic and Bit Operations/Compare To Zero  relop===  OutDataTypeStr=boolean  ZeroCross=off
  PhaseA_Ref : Sin  Amplitude=ma  Frequency=ref_frequency  SampleTime=0
  PhaseB_Ref : Sin  Amplitude=ma  Frequency=ref_frequency  Phase=-2*pi/3  SampleTime=0
  PhaseC_Ref : Sin  Amplitude=ma  Frequency=ref_frequency  Phase=2*pi/3  SampleTime=0
  Sum1 : Sum  Inputs=|+-
  Sum2 : Sum  Inputs=|+-
  Sum3 : Sum  Inputs=|+-
  Gate signals : Outport
  wires:
  Carrier_signal/1 -> [Carrier]
  Compare To Zero5/1 -> Bus Creator/6
  Compare To Zero4/1 -> Bus Creator/4
  Compare To Zero3/1 -> Bus Creator/2
  Sum3/1 -> Compare To Zero2/1
  Sum1/1 -> Compare To Zero1/1
  [Carrier] -> Sum3/2
  PhaseC_Ref/1 -> Sum3/1
  Compare To Zero2/1 -> Bus Creator/5, Compare To Zero5/1
  [Carrier] -> Sum1/2
  PhaseB_Ref/1 -> Sum1/1
  Compare To Zero1/1 -> Bus Creator/3, Compare To Zero4/1
  [Carrier] -> Sum2/2
  Sum2/1 -> Compare To Zero/1
  Compare To Zero/1 -> Bus Creator/1, Compare To Zero3/1
  PhaseA_Ref/1 -> Sum2/1
  Bus Creator/1 -> Gate signals/1

== system twolevel_seriesparallel/GateDrive8 ==
  Bus Creator : BusCreator  Inputs=6
  Carrier_signal : powerlib_meascontrol/Pulse & Signal Generators/Sawtooth Generator  Freq=sw_frequency  Phase=intangle8  Ts=0
  Compare To Zero : simulink/Logic and Bit Operations/Compare To Zero  relop=<=  OutDataTypeStr=boolean  ZeroCross=off
  Compare To Zero1 : simulink/Logic and Bit Operations/Compare To Zero  relop=<=  OutDataTypeStr=boolean  ZeroCross=off
  Compare To Zero2 : simulink/Logic and Bit Operations/Compare To Zero  relop=<=  OutDataTypeStr=boolean  ZeroCross=off
  Compare To Zero3 : simulink/Logic and Bit Operations/Compare To Zero  relop===  OutDataTypeStr=boolean  ZeroCross=off
  Compare To Zero4 : simulink/Logic and Bit Operations/Compare To Zero  relop===  OutDataTypeStr=boolean  ZeroCross=off
  Compare To Zero5 : simulink/Logic and Bit Operations/Compare To Zero  relop===  OutDataTypeStr=boolean  ZeroCross=off
  PhaseA_Ref : Sin  Amplitude=ma  Frequency=ref_frequency  SampleTime=0
  PhaseB_Ref : Sin  Amplitude=ma  Frequency=ref_frequency  Phase=-2*pi/3  SampleTime=0
  PhaseC_Ref : Sin  Amplitude=ma  Frequency=ref_frequency  Phase=2*pi/3  SampleTime=0
  Sum1 : Sum  Inputs=|+-
  Sum2 : Sum  Inputs=|+-
  Sum3 : Sum  Inputs=|+-
  Gate signals : Outport
  wires:
  Bus Creator/1 -> Gate signals/1
  PhaseA_Ref/1 -> Sum2/1
  Compare To Zero/1 -> Compare To Zero3/1, Bus Creator/1
  Sum2/1 -> Compare To Zero/1
  [Carrier] -> Sum2/2
  Compare To Zero1/1 -> Compare To Zero4/1, Bus Creator/3
  PhaseB_Ref/1 -> Sum1/1
  [Carrier] -> Sum1/2
  Compare To Zero2/1 -> Compare To Zero5/1, Bus Creator/5
  PhaseC_Ref/1 -> Sum3/1
  [Carrier] -> Sum3/2
  Sum1/1 -> Compare To Zero1/1
  Sum3/1 -> Compare To Zero2/1
  Compare To Zero3/1 -> Bus Creator/2
  Compare To Zero4/1 -> Bus Creator/4
  Compare To Zero5/1 -> Bus Creator/6
  Carrier_signal/1 -> [Carrier]

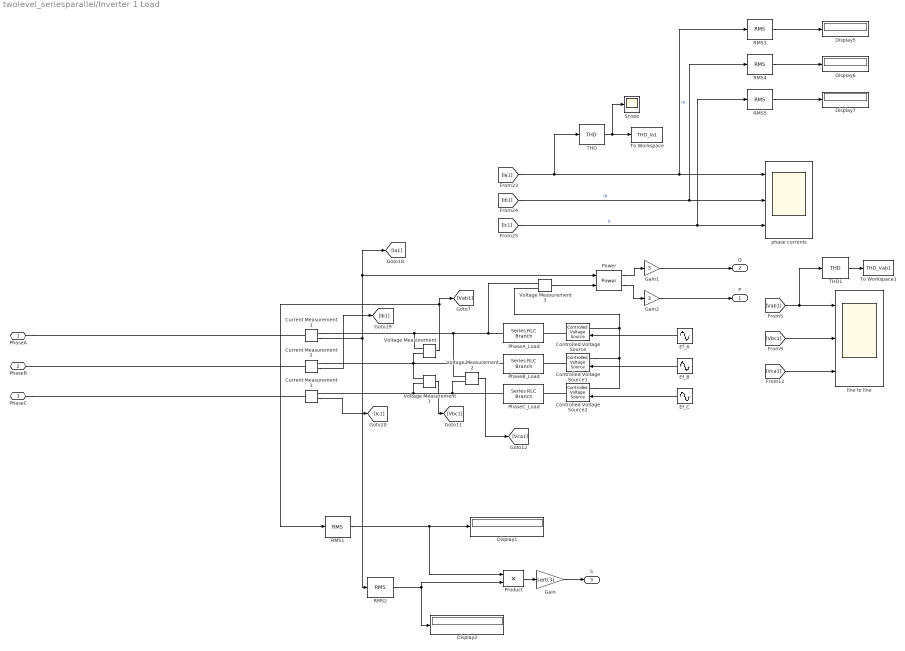
== system twolevel_seriesparallel/Inverter 1 Load ==
  Controlled Voltage Source : powerlib/Electrical Sources/Controlled Voltage Source  Initialize=on  Source_Type=AC  Amplitude=0  Phase=0  Frequency=0  Measurements=None
  Controlled Voltage Source1 : powerlib/Electrical Sources/Controlled Voltage Source  Initialize=on  Source_Type=AC  Amplitude=0  Phase=0  Frequency=0  Measurements=None
  Controlled Voltage Source2 : powerlib/Electrical Sources/Controlled Voltage Source  Initialize=on  Source_Type=AC  Amplitude=0  Phase=0  Frequency=0  Measurements=None
  Current Measurement1 : powerlib/Measurements/Current Measurement  PhasorSimulation=off  OutputType=Complex  PSBequivalent=0
  Current Measurement2 : powerlib/Measurements/Current Measurement  PhasorSimulation=off  OutputType=Complex  PSBequivalent=0
  Current Measurement3 : powerlib/Measurements/Current Measurement  PhasorSimulation=off  OutputType=Complex  PSBequivalent=0
  Display{1..2,5..7} (5 alike) : Display
  Ef_A : Sin  Amplitude=Ef*sqrt(2)  Frequency=ref_frequency  SampleTime=0
  Ef_B : Sin  Amplitude=Ef*sqrt(2)  Frequency=ref_frequency  Phase=-2*pi/3  SampleTime=0
  Ef_C : Sin  Amplitude=Ef*sqrt(2)  Frequency=ref_frequency  Phase=2*pi/3  SampleTime=0
  Gain : Gain  Gain=sqrt(3)
  Gain1 : Gain  Gain=3
  Gain2 : Gain  Gain=3
  PhaseA_Load : powerlib/Elements/Series RLC Branch  LConnTagsString=__new0  RConnTagsString=__new0  BranchType=L  Resistance=Rload  Inductance=Ls  SetiL0=off  InitialCurrent=0  Capacitance=1e-6  Setx0=off  InitialVoltage=0  Measurements=None
  PhaseB_Load : powerlib/Elements/Series RLC Branch  LConnTagsString=__new0  RConnTagsString=__new0  BranchType=L  Resistance=Rload  Inductance=Ls  SetiL0=off  InitialCurrent=0  Capacitance=1e-6  Setx0=off  InitialVoltage=0  Measurements=None
  PhaseC_Load : powerlib/Elements/Series RLC Branch  LConnTagsString=__new0  RConnTagsString=__new0  BranchType=L  Resistance=Rload  Inductance=Ls  SetiL0=off  InitialCurrent=0  Capacitance=1e-6  Setx0=off  InitialVoltage=0  Measurements=None
  Power : powerlib_meascontrol/Measurements/Power  Freq=50  Vinit=[1, 0]  Iinit=[1, 0]  Ts=0
  Product : Product
  RMS1 : powerlib_meascontrol/Measurements/RMS  TrueRMS=off  Freq=Load_Nominal_Freq  RMSInit=120  Ts=0
  RMS{2..5} (4 alike) : powerlib_meascontrol/Measurements/RMS  TrueRMS=on  Freq=Load_Nominal_Freq  RMSInit=120  Ts=0
  Scope : Scope
  THD : powerlib_meascontrol/Measurements/THD  Freq=50  Ts=0
  THD1 : powerlib_meascontrol/Measurements/THD  Freq=50  Ts=0
  To Workspace : ToWorkspace  VariableName=THD_Ia1  SaveFormat=Timeseries  SampleTime=-1
  To Workspace1 : ToWorkspace  VariableName=THD_Vab1  SaveFormat=Timeseries  SampleTime=-1
  Voltage Measurement{,1..3} (4 alike) : powerlib/Measurements/Voltage Measurement  PhasorSimulation=off  OutputType=Complex  PSBequivalent=0
  line to line : Scope  NumInputPorts=3
  phase currents : Scope  NumInputPorts=3
  PhaseA : PMIOPort  Port=1  Side=Left
  PhaseB : PMIOPort  Port=2  Side=Left
  PhaseC : PMIOPort  Port=3  Side=Left
  P : Outport
  Q : Outport  Port=2
  S : Outport  Port=3
  wires:
  Ef_C/1 -> Controlled Voltage Source2/1
  Ef_B/1 -> Controlled Voltage Source1/1
  Ef_A/1 -> Controlled Voltage Source/1
  Current Measurement1/1 -> RMS2/1, Power/2, [Ia1]
  RMS5/1 -> Display7/1
  RMS4/1 -> Display6/1
  RMS3/1 -> Display5/1
  Gain2/1 -> P/1
  Gain1/1 -> Q/1
  Voltage Measurement3/1 -> Power/1
  Power/1 -> Gain2/1
  Power/2 -> Gain1/1
  Gain/1 -> S/1
  RMS2/1 -> Display2/1, Product/2
  RMS1/1 -> Display1/1, Product/1
  Product/1 -> Gain/1
  THD1/1 -> To Workspace1/1
  [Ib1] -> phase currents/2, RMS4/1  "Ib"
  Voltage Measurement2/1 -> [Vca1]
  THD/1 -> Scope/1, To Workspace/1
  [Vca1] -> line to line/3
  [Vab1] -> line to line/1, THD1/1
  [Vbc1] -> line to line/2
  [Ic1] -> phase currents/3, RMS5/1  "Ic"
  [Ia1] -> phase currents/1, RMS3/1, THD/1  "Ia"
  Current Measurement3/1 -> [Ic1]
  Voltage Measurement1/1 -> [Vbc1]
  Voltage Measurement/1 -> RMS1/1, [Vab1]
  Current Measurement2/1 -> [Ib1]
  connections:
  Controlled Voltage Source2/RConn1 -- PhaseC_Load/RConn1
  Controlled Voltage Source/RConn1 -- PhaseA_Load/RConn1
  Controlled Voltage Source1/RConn1 -- PhaseB_Load/RConn1
  Controlled Voltage Source/LConn1 -- Voltage Measurement3/LConn2 -- Controlled Voltage Source1/LConn1 -- Controlled Voltage Source2/LConn1
  PhaseA_Load/LConn1 -- Voltage Measurement3/LConn1 -- Voltage Measurement2/LConn2 -- Voltage Measurement/LConn1 -- Current Measurement1/RConn1
  PhaseA/RConn1 -- Current Measurement1/LConn1
  Current Measurement2/LConn1 -- PhaseB/RConn1
  Current Measurement3/RConn1 -- Voltage Measurement1/LConn2 -- Voltage Measurement2/LConn1 -- PhaseC_Load/LConn1
  PhaseC/RConn1 -- Current Measurement3/LConn1
  PhaseB_Load/LConn1 -- Voltage Measurement/LConn2 -- Voltage Measurement1/LConn1 -- Current Measurement2/RConn1

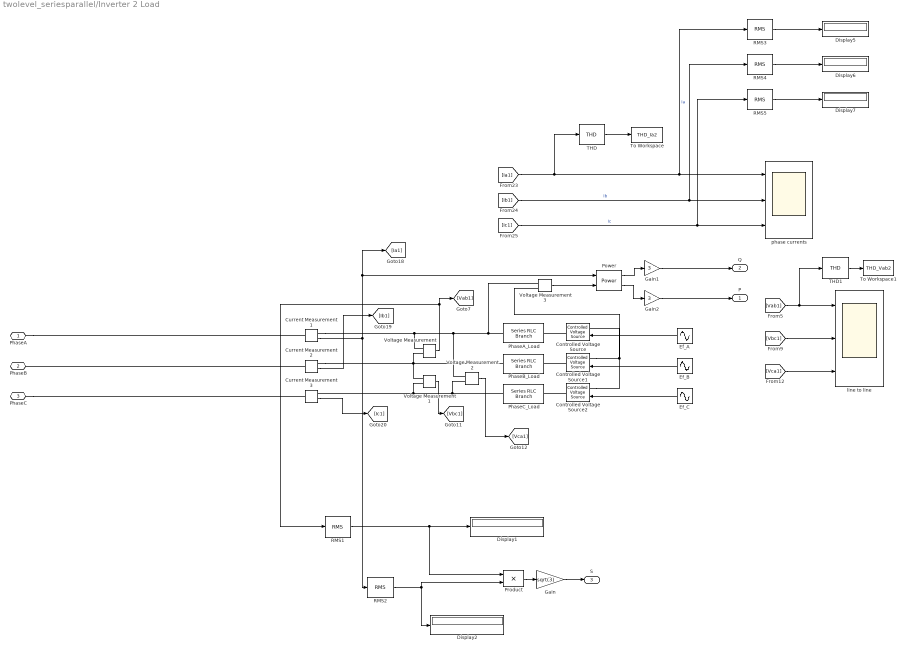
== system twolevel_seriesparallel/Inverter 2 Load ==
  Controlled Voltage Source : powerlib/Electrical Sources/Controlled Voltage Source  Initialize=on  Source_Type=AC  Amplitude=0  Phase=0  Frequency=0  Measurements=None
  Controlled Voltage Source1 : powerlib/Electrical Sources/Controlled Voltage Source  Initialize=on  Source_Type=AC  Amplitude=0  Phase=0  Frequency=0  Measurements=None
  Controlled Voltage Source2 : powerlib/Electrical Sources/Controlled Voltage Source  Initialize=on  Source_Type=AC  Amplitude=0  Phase=0  Frequency=0  Measurements=None
  Current Measurement1 : powerlib/Measurements/Current Measurement  PhasorSimulation=off  OutputType=Complex  PSBequivalent=0
  Current Measurement2 : powerlib/Measurements/Current Measurement  PhasorSimulation=off  OutputType=Complex  PSBequivalent=0
  Current Measurement3 : powerlib/Measurements/Current Measurement  PhasorSimulation=off  OutputType=Complex  PSBequivalent=0
  Display{1..2,5..7} (5 alike) : Display
  Ef_A : Sin  Amplitude=Ef*sqrt(2)  Frequency=ref_frequency  SampleTime=0
  Ef_B : Sin  Amplitude=Ef*sqrt(2)  Frequency=ref_frequency  Phase=-2*pi/3  SampleTime=0
  Ef_C : Sin  Amplitude=Ef*sqrt(2)  Frequency=ref_frequency  Phase=2*pi/3  SampleTime=0
  Gain : Gain  Gain=sqrt(3)
  Gain1 : Gain  Gain=3
  Gain2 : Gain  Gain=3
  PhaseA_Load : powerlib/Elements/Series RLC Branch  LConnTagsString=__new0  RConnTagsString=__new0  BranchType=L  Resistance=Rload  Inductance=Ls  SetiL0=off  InitialCurrent=0  Capacitance=1e-6  Setx0=off  InitialVoltage=0  Measurements=None
  PhaseB_Load : powerlib/Elements/Series RLC Branch  LConnTagsString=__new0  RConnTagsString=__new0  BranchType=L  Resistance=Rload  Inductance=Ls  SetiL0=off  InitialCurrent=0  Capacitance=1e-6  Setx0=off  InitialVoltage=0  Measurements=None
  PhaseC_Load : powerlib/Elements/Series RLC Branch  LConnTagsString=__new0  RConnTagsString=__new0  BranchType=L  Resistance=Rload  Inductance=Ls  SetiL0=off  InitialCurrent=0  Capacitance=1e-6  Setx0=off  InitialVoltage=0  Measurements=None
  Power : powerlib_meascontrol/Measurements/Power  Freq=50  Vinit=[1, 0]  Iinit=[1, 0]  Ts=0
  Product : Product
  RMS1 : powerlib_meascontrol/Measurements/RMS  TrueRMS=off  Freq=Load_Nominal_Freq  RMSInit=120  Ts=0
  RMS{2..5} (4 alike) : powerlib_meascontrol/Measurements/RMS  TrueRMS=on  Freq=Load_Nominal_Freq  RMSInit=120  Ts=0
  THD : powerlib_meascontrol/Measurements/THD  Freq=50  Ts=0
  THD1 : powerlib_meascontrol/Measurements/THD  Freq=50  Ts=0
  To Workspace : ToWorkspace  VariableName=THD_Ia2  SaveFormat=Timeseries  SampleTime=-1
  To Workspace1 : ToWorkspace  VariableName=THD_Vab2  SaveFormat=Timeseries  SampleTime=-1
  Voltage Measurement{,1..3} (4 alike) : powerlib/Measurements/Voltage Measurement  PhasorSimulation=off  OutputType=Complex  PSBequivalent=0
  line to line : Scope  NumInputPorts=3
  phase currents : Scope  NumInputPorts=3
  PhaseA : PMIOPort  Port=1  Side=Left
  PhaseB : PMIOPort  Port=2  Side=Left
  PhaseC : PMIOPort  Port=3  Side=Left
  P : Outport
  Q : Outport  Port=2
  S : Outport  Port=3
  wires:
  Current Measurement2/1 -> [Ib1]
  Voltage Measurement/1 -> [Vab1], RMS1/1
  Voltage Measurement1/1 -> [Vbc1]
  Current Measurement3/1 -> [Ic1]
  [Ia1] -> THD/1, RMS3/1, phase currents/1  "Ia"
  [Ic1] -> RMS5/1, phase currents/3  "Ic"
  [Vbc1] -> line to line/2
  [Vab1] -> THD1/1, line to line/1
  [Vca1] -> line to line/3
  THD/1 -> To Workspace/1
  Voltage Measurement2/1 -> [Vca1]
  [Ib1] -> RMS4/1, phase currents/2  "Ib"
  THD1/1 -> To Workspace1/1
  Product/1 -> Gain/1
  RMS1/1 -> Product/1, Display1/1
  RMS2/1 -> Product/2, Display2/1
  Gain/1 -> S/1
  Power/2 -> Gain1/1
  Power/1 -> Gain2/1
  Voltage Measurement3/1 -> Power/1
  Gain1/1 -> Q/1
  Gain2/1 -> P/1
  RMS3/1 -> Display5/1
  RMS4/1 -> Display6/1
  RMS5/1 -> Display7/1
  Current Measurement1/1 -> [Ia1], Power/2, RMS2/1
  Ef_A/1 -> Controlled Voltage Source/1
  Ef_B/1 -> Controlled Voltage Source1/1
  Ef_C/1 -> Controlled Voltage Source2/1
  connections:
  Current Measurement2/RConn1 -- Voltage Measurement1/LConn1 -- Voltage Measurement/LConn2 -- PhaseB_Load/LConn1
  PhaseC/RConn1 -- Current Measurement3/LConn1
  PhaseC_Load/LConn1 -- Voltage Measurement2/LConn1 -- Voltage Measurement1/LConn2 -- Current Measurement3/RConn1
  Current Measurement2/LConn1 -- PhaseB/RConn1
  PhaseA/RConn1 -- Current Measurement1/LConn1
  Current Measurement1/RConn1 -- Voltage Measurement/LConn1 -- Voltage Measurement2/LConn2 -- Voltage Measurement3/LConn1 -- PhaseA_Load/LConn1
  Controlled Voltage Source2/LConn1 -- Controlled Voltage Source1/LConn1 -- Voltage Measurement3/LConn2 -- Controlled Voltage Source/LConn1
  Controlled Voltage Source1/RConn1 -- PhaseB_Load/RConn1
  Controlled Voltage Source/RConn1 -- PhaseA_Load/RConn1
  Controlled Voltage Source2/RConn1 -- PhaseC_Load/RConn1

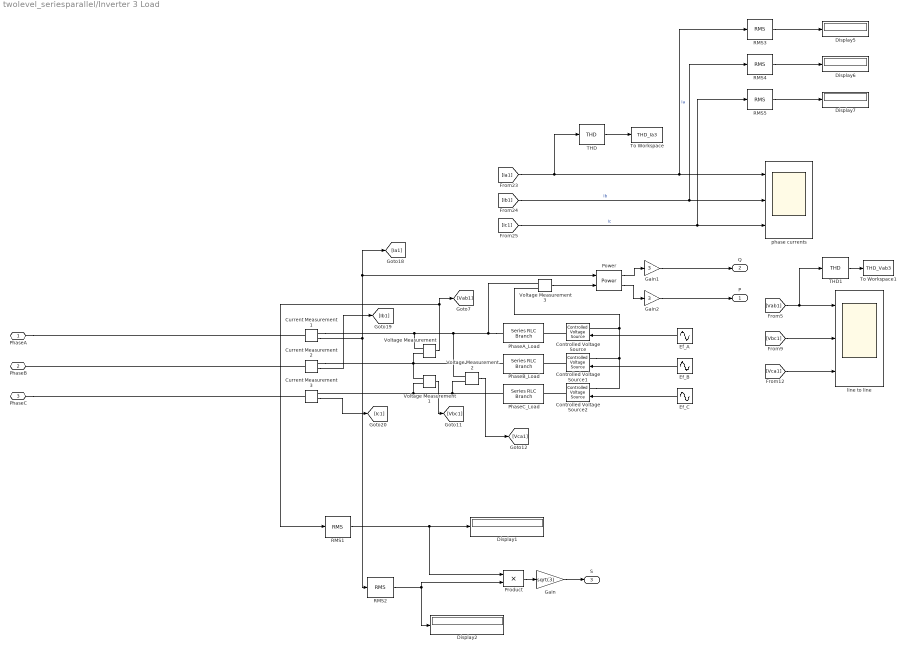
== system twolevel_seriesparallel/Inverter 3 Load ==
  Controlled Voltage Source : powerlib/Electrical Sources/Controlled Voltage Source  Initialize=on  Source_Type=AC  Amplitude=0  Phase=0  Frequency=0  Measurements=None
  Controlled Voltage Source1 : powerlib/Electrical Sources/Controlled Voltage Source  Initialize=on  Source_Type=AC  Amplitude=0  Phase=0  Frequency=0  Measurements=None
  Controlled Voltage Source2 : powerlib/Electrical Sources/Controlled Voltage Source  Initialize=on  Source_Type=AC  Amplitude=0  Phase=0  Frequency=0  Measurements=None
  Current Measurement1 : powerlib/Measurements/Current Measurement  PhasorSimulation=off  OutputType=Complex  PSBequivalent=0
  Current Measurement2 : powerlib/Measurements/Current Measurement  PhasorSimulation=off  OutputType=Complex  PSBequivalent=0
  Current Measurement3 : powerlib/Measurements/Current Measurement  PhasorSimulation=off  OutputType=Complex  PSBequivalent=0
  Display{1..2,5..7} (5 alike) : Display
  Ef_A : Sin  Amplitude=Ef*sqrt(2)  Frequency=ref_frequency  SampleTime=0
  Ef_B : Sin  Amplitude=Ef*sqrt(2)  Frequency=ref_frequency  Phase=-2*pi/3  SampleTime=0
  Ef_C : Sin  Amplitude=Ef*sqrt(2)  Frequency=ref_frequency  Phase=2*pi/3  SampleTime=0
  Gain : Gain  Gain=sqrt(3)
  Gain1 : Gain  Gain=3
  Gain2 : Gain  Gain=3
  PhaseA_Load : powerlib/Elements/Series RLC Branch  LConnTagsString=__new0  RConnTagsString=__new0  BranchType=L  Resistance=Rload  Inductance=Ls  SetiL0=off  InitialCurrent=0  Capacitance=1e-6  Setx0=off  InitialVoltage=0  Measurements=None
  PhaseB_Load : powerlib/Elements/Series RLC Branch  LConnTagsString=__new0  RConnTagsString=__new0  BranchType=L  Resistance=Rload  Inductance=Ls  SetiL0=off  InitialCurrent=0  Capacitance=1e-6  Setx0=off  InitialVoltage=0  Measurements=None
  PhaseC_Load : powerlib/Elements/Series RLC Branch  LConnTagsString=__new0  RConnTagsString=__new0  BranchType=L  Resistance=Rload  Inductance=Ls  SetiL0=off  InitialCurrent=0  Capacitance=1e-6  Setx0=off  InitialVoltage=0  Measurements=None
  Power : powerlib_meascontrol/Measurements/Power  Freq=50  Vinit=[1, 0]  Iinit=[1, 0]  Ts=0
  Product : Product
  RMS1 : powerlib_meascontrol/Measurements/RMS  TrueRMS=off  Freq=Load_Nominal_Freq  RMSInit=120  Ts=0
  RMS{2..5} (4 alike) : powerlib_meascontrol/Measurements/RMS  TrueRMS=on  Freq=Load_Nominal_Freq  RMSInit=120  Ts=0
  THD : powerlib_meascontrol/Measurements/THD  Freq=50  Ts=0
  THD1 : powerlib_meascontrol/Measurements/THD  Freq=50  Ts=0
  To Workspace : ToWorkspace  VariableName=THD_Ia3  SaveFormat=Timeseries  SampleTime=-1
  To Workspace1 : ToWorkspace  VariableName=THD_Vab3  SaveFormat=Timeseries  SampleTime=-1
  Voltage Measurement{,1..3} (4 alike) : powerlib/Measurements/Voltage Measurement  PhasorSimulation=off  OutputType=Complex  PSBequivalent=0
  line to line : Scope  NumInputPorts=3
  phase currents : Scope  NumInputPorts=3
  PhaseA : PMIOPort  Port=1  Side=Left
  PhaseB : PMIOPort  Port=2  Side=Left
  PhaseC : PMIOPort  Port=3  Side=Left
  P : Outport
  Q : Outport  Port=2
  S : Outport  Port=3
  wires:
  Ef_C/1 -> Controlled Voltage Source2/1
  Ef_B/1 -> Controlled Voltage Source1/1
  Ef_A/1 -> Controlled Voltage Source/1
  Current Measurement1/1 -> RMS2/1, Power/2, [Ia1]
  RMS5/1 -> Display7/1
  RMS4/1 -> Display6/1
  RMS3/1 -> Display5/1
  Gain2/1 -> P/1
  Gain1/1 -> Q/1
  Voltage Measurement3/1 -> Power/1
  Power/1 -> Gain2/1
  Power/2 -> Gain1/1
  Gain/1 -> S/1
  RMS2/1 -> Display2/1, Product/2
  RMS1/1 -> Display1/1, Product/1
  Product/1 -> Gain/1
  THD1/1 -> To Workspace1/1
  [Ib1] -> phase currents/2, RMS4/1  "Ib"
  Voltage Measurement2/1 -> [Vca1]
  THD/1 -> To Workspace/1
  [Vca1] -> line to line/3
  [Vab1] -> line to line/1, THD1/1
  [Vbc1] -> line to line/2
  [Ic1] -> phase currents/3, RMS5/1  "Ic"
  [Ia1] -> phase currents/1, RMS3/1, THD/1  "Ia"
  Current Measurement3/1 -> [Ic1]
  Voltage Measurement1/1 -> [Vbc1]
  Voltage Measurement/1 -> RMS1/1, [Vab1]
  Current Measurement2/1 -> [Ib1]
  connections:
  Controlled Voltage Source2/RConn1 -- PhaseC_Load/RConn1
  Controlled Voltage Source/RConn1 -- PhaseA_Load/RConn1
  Controlled Voltage Source1/RConn1 -- PhaseB_Load/RConn1
  Controlled Voltage Source/LConn1 -- Voltage Measurement3/LConn2 -- Controlled Voltage Source1/LConn1 -- Controlled Voltage Source2/LConn1
  PhaseA_Load/LConn1 -- Voltage Measurement3/LConn1 -- Voltage Measurement2/LConn2 -- Voltage Measurement/LConn1 -- Current Measurement1/RConn1
  PhaseA/RConn1 -- Current Measurement1/LConn1
  Current Measurement2/LConn1 -- PhaseB/RConn1
  Current Measurement3/RConn1 -- Voltage Measurement1/LConn2 -- Voltage Measurement2/LConn1 -- PhaseC_Load/LConn1
  PhaseC/RConn1 -- Current Measurement3/LConn1
  PhaseB_Load/LConn1 -- Voltage Measurement/LConn2 -- Voltage Measurement1/LConn1 -- Current Measurement2/RConn1

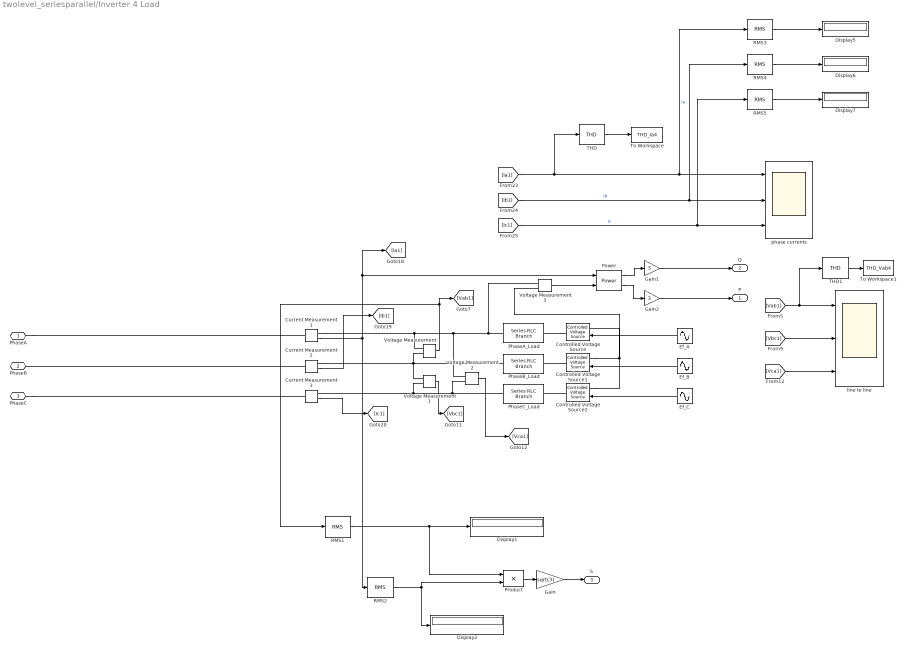
== system twolevel_seriesparallel/Inverter 4 Load ==
  Controlled Voltage Source : powerlib/Electrical Sources/Controlled Voltage Source  Initialize=on  Source_Type=AC  Amplitude=0  Phase=0  Frequency=0  Measurements=None
  Controlled Voltage Source1 : powerlib/Electrical Sources/Controlled Voltage Source  Initialize=on  Source_Type=AC  Amplitude=0  Phase=0  Frequency=0  Measurements=None
  Controlled Voltage Source2 : powerlib/Electrical Sources/Controlled Voltage Source  Initialize=on  Source_Type=AC  Amplitude=0  Phase=0  Frequency=0  Measurements=None
  Current Measurement1 : powerlib/Measurements/Current Measurement  PhasorSimulation=off  OutputType=Complex  PSBequivalent=0
  Current Measurement2 : powerlib/Measurements/Current Measurement  PhasorSimulation=off  OutputType=Complex  PSBequivalent=0
  Current Measurement3 : powerlib/Measurements/Current Measurement  PhasorSimulation=off  OutputType=Complex  PSBequivalent=0
  Display{1..2,5..7} (5 alike) : Display
  Ef_A : Sin  Amplitude=Ef*sqrt(2)  Frequency=ref_frequency  SampleTime=0
  Ef_B : Sin  Amplitude=Ef*sqrt(2)  Frequency=ref_frequency  Phase=-2*pi/3  SampleTime=0
  Ef_C : Sin  Amplitude=Ef*sqrt(2)  Frequency=ref_frequency  Phase=2*pi/3  SampleTime=0
  Gain : Gain  Gain=sqrt(3)
  Gain1 : Gain  Gain=3
  Gain2 : Gain  Gain=3
  PhaseA_Load : powerlib/Elements/Series RLC Branch  LConnTagsString=__new0  RConnTagsString=__new0  BranchType=L  Resistance=Rload  Inductance=Ls  SetiL0=off  InitialCurrent=0  Capacitance=1e-6  Setx0=off  InitialVoltage=0  Measurements=None
  PhaseB_Load : powerlib/Elements/Series RLC Branch  LConnTagsString=__new0  RConnTagsString=__new0  BranchType=L  Resistance=Rload  Inductance=Ls  SetiL0=off  InitialCurrent=0  Capacitance=1e-6  Setx0=off  InitialVoltage=0  Measurements=None
  PhaseC_Load : powerlib/Elements/Series RLC Branch  LConnTagsString=__new0  RConnTagsString=__new0  BranchType=L  Resistance=Rload  Inductance=Ls  SetiL0=off  InitialCurrent=0  Capacitance=1e-6  Setx0=off  InitialVoltage=0  Measurements=None
  Power : powerlib_meascontrol/Measurements/Power  Freq=50  Vinit=[1, 0]  Iinit=[1, 0]  Ts=0
  Product : Product
  RMS1 : powerlib_meascontrol/Measurements/RMS  TrueRMS=off  Freq=Load_Nominal_Freq  RMSInit=120  Ts=0
  RMS{2..5} (4 alike) : powerlib_meascontrol/Measurements/RMS  TrueRMS=on  Freq=Load_Nominal_Freq  RMSInit=120  Ts=0
  THD : powerlib_meascontrol/Measurements/THD  Freq=50  Ts=0
  THD1 : powerlib_meascontrol/Measurements/THD  Freq=50  Ts=0
  To Workspace : ToWorkspace  VariableName=THD_Ia4  SaveFormat=Timeseries  SampleTime=-1
  To Workspace1 : ToWorkspace  VariableName=THD_Vab4  SaveFormat=Timeseries  SampleTime=-1
  Voltage Measurement{,1..3} (4 alike) : powerlib/Measurements/Voltage Measurement  PhasorSimulation=off  OutputType=Complex  PSBequivalent=0
  line to line : Scope  NumInputPorts=3
  phase currents : Scope  NumInputPorts=3
  PhaseA : PMIOPort  Port=1  Side=Left
  PhaseB : PMIOPort  Port=2  Side=Left
  PhaseC : PMIOPort  Port=3  Side=Left
  P : Outport
  Q : Outport  Port=2
  S : Outport  Port=3
  wires:
  Current Measurement2/1 -> [Ib1]
  Voltage Measurement/1 -> [Vab1], RMS1/1
  Voltage Measurement1/1 -> [Vbc1]
  Current Measurement3/1 -> [Ic1]
  [Ia1] -> THD/1, RMS3/1, phase currents/1  "Ia"
  [Ic1] -> RMS5/1, phase currents/3  "Ic"
  [Vbc1] -> line to line/2
  [Vab1] -> THD1/1, line to line/1
  [Vca1] -> line to line/3
  THD/1 -> To Workspace/1
  Voltage Measurement2/1 -> [Vca1]
  [Ib1] -> RMS4/1, phase currents/2  "Ib"
  THD1/1 -> To Workspace1/1
  Product/1 -> Gain/1
  RMS1/1 -> Product/1, Display1/1
  RMS2/1 -> Product/2, Display2/1
  Gain/1 -> S/1
  Power/2 -> Gain1/1
  Power/1 -> Gain2/1
  Voltage Measurement3/1 -> Power/1
  Gain1/1 -> Q/1
  Gain2/1 -> P/1
  RMS3/1 -> Display5/1
  RMS4/1 -> Display6/1
  RMS5/1 -> Display7/1
  Current Measurement1/1 -> [Ia1], Power/2, RMS2/1
  Ef_A/1 -> Controlled Voltage Source/1
  Ef_B/1 -> Controlled Voltage Source1/1
  Ef_C/1 -> Controlled Voltage Source2/1
  connections:
  Current Measurement2/RConn1 -- Voltage Measurement1/LConn1 -- Voltage Measurement/LConn2 -- PhaseB_Load/LConn1
  PhaseC/RConn1 -- Current Measurement3/LConn1
  PhaseC_Load/LConn1 -- Voltage Measurement2/LConn1 -- Voltage Measurement1/LConn2 -- Current Measurement3/RConn1
  Current Measurement2/LConn1 -- PhaseB/RConn1
  PhaseA/RConn1 -- Current Measurement1/LConn1
  Current Measurement1/RConn1 -- Voltage Measurement/LConn1 -- Voltage Measurement2/LConn2 -- Voltage Measurement3/LConn1 -- PhaseA_Load/LConn1
  Controlled Voltage Source2/LConn1 -- Controlled Voltage Source1/LConn1 -- Voltage Measurement3/LConn2 -- Controlled Voltage Source/LConn1
  Controlled Voltage Source1/RConn1 -- PhaseB_Load/RConn1
  Controlled Voltage Source/RConn1 -- PhaseA_Load/RConn1
  Controlled Voltage Source2/RConn1 -- PhaseC_Load/RConn1
